simulink model "Question2_simulink"  (R2017b)
settings: Solver=FixedStepAuto  StartTime=0.0  StopTime=1  FixedStep=.0001  RelTol=1e-3
values from neighbouring files (symbols this model uses):
  Kt = 0.3    [Question_2_code.m]
  Tem_final = 9    [Question_2_code.m]
  Tem_initial = 6    [Question_2_code.m]
settings Model: Creator=Andrew McCullough  LastModifiedBy=Andrew McCullough

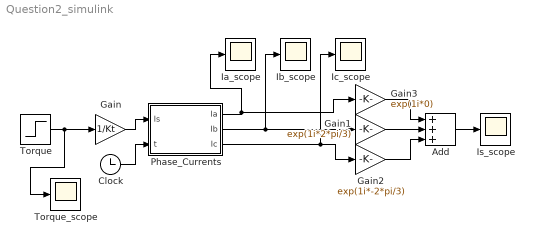
== system Question2_simulink ==
  Add : Sum  Inputs=+++
  Clock : Clock
  Gain : Gain  Gain=1/Kt
  Gain1 : Gain  Gain=exp(1i*2*pi/3)
  Gain2 : Gain  Gain=exp(1i*-2*pi/3)
  Gain3 : Gain  Gain=exp(1i*0)
  Ia_scope : Scope
  Ib_scope : Scope
  Ic_scope : Scope
  Is_scope : Scope
  Phase_Currents : MATLAB Function  TreatAsAtomicUnit=on
  Torque : Step  Time=.3  Before=Tem_initial  After=Tem_final  SampleTime=0
  Torque_scope : Scope
  wires:
  Torque/1 -> Gain/1, Torque_scope/1
  Gain/1 -> Phase_Currents/1(Is)
  Add/1 -> Is_scope/1
  Phase_Currents/2(Ib) -> Gain1/1, Ib_scope/1
  Phase_Currents/1(Ia) -> Gain3/1, Ia_scope/1
  Phase_Currents/3(Ic) -> Gain2/1, Ic_scope/1
  Clock/1 -> Phase_Currents/2(t)
  Gain3/1 -> Add/1
  Gain1/1 -> Add/2
  Gain2/1 -> Add/3

== matlab function Question2_simulink/Phase_Currents ==
  data: Ia output; Ib output; Is input; Ic output; t input
function [Ia, Ib, Ic]= fcn(Is,t)

w = 2*pi*60;
Is = Is*exp(1i*w*t);

Ia = (2/3)*real(Is*exp(1i*0));
Ib = (2/3)*real(Is*exp(1i*((-2*pi)/3)));
Ic = (2/3)*real(Is*exp(1i*((-4*pi)/3)));
